simulink library "dotFinder_ul"  (R2018b)
settings: Solver=VariableStepAuto  StartTime=0.0  StopTime=10.0  RelTol=1e-3
libraries: simulink x2
settings Model: Creator=mcobb  LastModifiedBy=mcobb
settings DebuggingCC: LibraryContextMissingDiagnostic=none
settings SFSimCC: SimUseLocalCustomCode=off
settings RTWCC: RTWUseLocalCustomCode=off

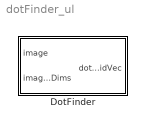
== system dotFinder_ul ==
  DotFinder : Subsystem  mask{ROIPositionHoldEnable=on, ROIPositionHoldCoordinates=1*[500 500], ROIDimVec_px=[40 100], ImageDimensions=[1000 2000]}
      mask prompts: ROIPositionHoldEnable "Hold Position Enable"; ROIPositionHoldCoordinates "Hold Position Coordinates  [rows cols]  (pixels)"; ROIDimVec_px "Dimensions [rows cols]  (pixels)"; ImageDimensions "Image Dimensions [rows cols] in pixels"
      mask DialogControl ParameterGroupVar Prompt: Region Of Interest (ROI) Parameters
      mask DialogControl Container3 Prompt: Other Parameters

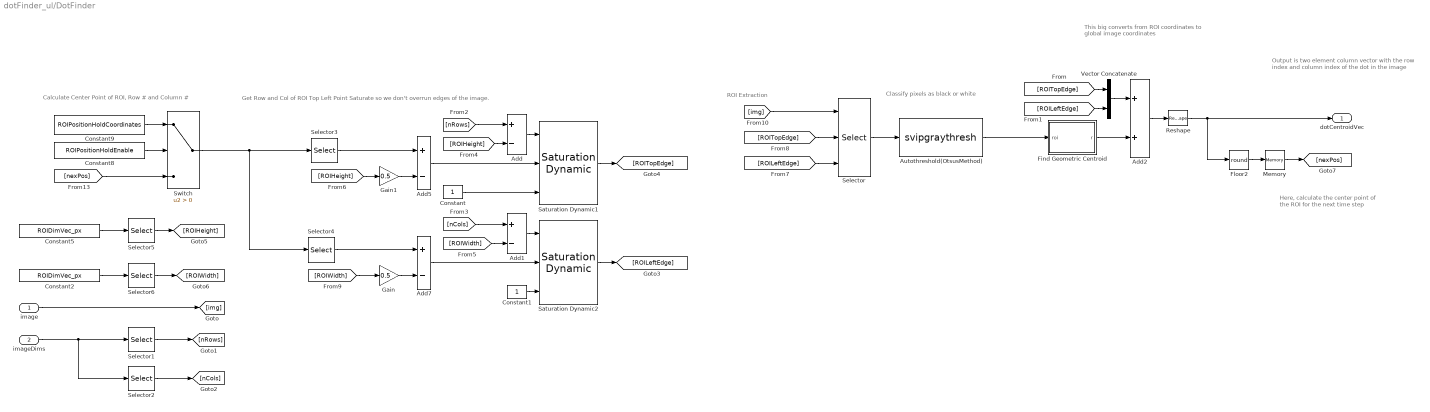
== system dotFinder_ul/DotFinder ==
  note: This big converts from ROI coordinates
      | to global image coordinates
  note: Here, calculate the center point of
      | the ROI for the next time step
  note: Output is two element column vector with the row
      | index and column index of the dot in the image
  note: Classify pixels as black or white
  note: Get Row and Col of ROI Top Left Point
      | Saturate so we don't overrun edges of the image.
  note: Calculate Center Point of ROI, Row # and Column #
  note: ROI Extraction
  image : Inport
  imageDims : Inport  Port=2
  Add{,1,5,7} (4 alike) : Sum  Inputs=+-
  Add2 : Sum
  Autothreshold(OtsusMethod) : S-Function  DialogController=vipDDGCreate  FunctionName=svipgraythresh  Parameters=operator, userDefinedRange, umin, umax, threshOut, effMetricOut, outOfRngOpt, scaleThreshold, scaleFactor, P1Mode, P1WordLength, P1FracLength, A1Mode, A1WordLength, A1FracLength, P2Mode, P2WordLength, P2FracLength, A2Mode, A2WordLength, A2FracLength, P3Mode, P3WordLength, P3FracLength, A3Mode, A3WordLength, A3FracLength, P4Mode, P4WordLength, P4FracLength, A4Mode, A4WordLength, A4FracLength, Q1Mode, Q1WordLength, Q1FracLength, EMMode, EMWordLength, EMFracLength, dtInfo.roundingMode, dtInfo.overflowMode  SFunctionDeploymentMode=off  EnableBusSupport=off  mask(Autothreshold){operator=>, threshOut=off, effMetricOut=off, userDefinedRange=off, umin=0, umax=255, outOfRngOpt=Ignore, scaleThreshold=off, scaleFactor=1, P1Mode=Specify word length, P1WordLength=32, P1FracLength=30, A1Mode=Same as Product 1, A1WordLength=32, A1FracLength=30, P2Mode=Specify word length, P2WordLength=32, P2FracLength=22, A2Mode=Same as Product 2, A2WordLength=32, A2FracLength=22, P3Mode=Specify word length, P3WordLength=32, P3FracLength=14, A3Mode=Same as Product 3, A3WordLength=32, A3FracLength=14, P4Mode=Binary point scaling, P4WordLength=32, P4FracLength=15, A4Mode=Same as Product 4, A4WordLength=16, A4FracLength=4, Q1Mode=Specify word length, Q1WordLength=32, Q1FracLength=16, EMMode=Specify word length, EMWordLength=16, EMFracLength=14, roundingMode=Floor, overflowMode=off, LockScale=off}
      mask prompts: operator "vision:masks:ThresholdingOperator"; threshOut "vision:masks:OutputThreshold"; effMetricOut "vision:masks:OutputEffectivenessMetric"; userDefinedRange "vision:masks:SpecifyDataRange"; umin "vision:masks:MinimumValueOfInput"; umax "vision:masks:MinimumValueOfInput"; outOfRngOpt "vision:masks:WhenDataRangeIsExceeded"; scaleThreshold "vision:masks:ScaleThreshold_MP"; scaleFactor "vision:masks:ThresholdScalingFactor"; P1Mode "P1:"; P1WordLength "P1 WL:"; P1FracLength "P1 FL:"; A1Mode "A1:"; A1WordLength "A1 WL:"; A1FracLength "A1 FL:"; P2Mode "P2:"; P2WordLength "P2 WL:"; P2FracLength "P2 FL:"; A2Mode "A2:"; A2WordLength "A2 WL:"; A2FracLength "A2 FL:"; P3Mode "P3:"; P3WordLength "P3 WL:"; P3FracLength "P3 FL:"; A3Mode "A3:"; A3WordLength "A3 WL:"; A3FracLength "A3 FL:"; P4Mode "P4:"; P4WordLength "P4 WL:"; P4FracLength "P4 FL:"; A4Mode "A4:"; A4WordLength "A4 WL:"; A4FracLength "A4 FL:"; Q1Mode "Q1:"; Q1WordLength "Q1 WL:"; Q1FracLength "Q1 FL:"; EMMode "EM:"; EMWordLength "EM WL:"; EMFracLength "EM FL:"; roundingMode "vision:masks:RoundIntegerCalculationsTowards"; overflowMode "vision:masks:RoundIntegerCalculationsTowards"; LockScale "vision:masks:LockScaling"
      mask help: vision:masks:AutoThresholdDescription
      mask init:
      | blk = gcbh;
      | 
      | dtInfo = dspGetFixptDataTypeInfo(blk,1);
      | 
      | effMetricOut_str = get_param(blk,'effMetricOut');
      | threshOut_str = get_param(blk,'threshOut');
      | if strcmp(effMetricOut_str,'off') && strcmp(threshOut_str,'off')
      | 	[so(1:3).port] = deal(1,1,1);
      | 	[so(1:3).txt] = deal('BW','BW','BW');
      | elseif strcmp(effMetricOut_str,'on') && strcmp(threshOut_str,'off')
      | 	[so(1:3).port] = deal(1,2,2);
      | 	[so(1:3).txt] = deal('BW','EMetric','EMetric');
      | elseif strcmp(effMetricOut_str,'off') && strcmp(threshOut_str,'on')
      | 	[so(1:3).port] = deal(1,2,2);
      | 	[so(1:3).txt] = deal('BW','Th','Th');
      | else
      | 	[so(1:3).port] = deal(1,2,3);
      | 	[so(1:3).txt] = deal('BW','Th','EMetric');
      | end
      mask Help: eval('visionblockhelp');
      mask TypeOptions operator: > | <=
      mask TypeOptions outOfRngOpt: vision:masks:Ignore | vision:masks:Saturate | vision:masks:WarnAndSaturate | vision:masks:Error
      mask TypeOptions P1Mode: Specify word length | Binary point scaling | Slope and bias scaling
      mask TypeOptions A1Mode: Same as Product 1 | Specify word length | Binary point scaling | Slope and bias scaling
      mask TypeOptions P2Mode: Specify word length | Binary point scaling | Slope and bias scaling
      mask TypeOptions A2Mode: Same as Product 2 | Specify word length | Binary point scaling | Slope and bias scaling
      mask TypeOptions P3Mode: Specify word length | Binary point scaling | Slope and bias scaling
      mask TypeOptions A3Mode: Same as Product 3 | Specify word length | Binary point scaling | Slope and bias scaling
      mask TypeOptions P4Mode: Same as input | Binary point scaling | Slope and bias scaling
      mask TypeOptions A4Mode: Same as Product 4 | Binary point scaling | Slope and bias scaling
      mask TypeOptions Q1Mode: Specify word length | Binary point scaling | Slope and bias scaling
      mask TypeOptions EMMode: Specify word length | Binary point scaling | Slope and bias scaling
      mask TypeOptions roundingMode: dspshared:FixptDialog:Ceiling_CB | dspshared:FixptDialog:Convergent_CB | dspshared:FixptDialog:Floor_CB | dspshared:FixptDialog:Nearest_CB | dspshared:FixptDialog:Round_CB | dspshared:FixptDialog:Simplest_CB | dspshared:FixptDialog:Zero_CB
      mask Display:
      | disp('Autothreshold');
      | port_label('input',1,'I');
      | port_label('output',so(1).port, so(1).txt);
      | port_label('output',so(2).port, so(2).txt);
      | port_label('output',so(3).port, so(3).txt);
  Constant : Constant
  Constant1 : Constant
  Constant2 : Constant  Value=ROIDimVec_px
  Constant5 : Constant  Value=ROIDimVec_px
  Constant8 : Constant  Value=ROIPositionHoldEnable
  Constant9 : Constant  Value=ROIPositionHoldCoordinates
  Find Geometric Centroid : MATLAB Function  TreatAsAtomicUnit=on
  Floor2 : Rounding  Operator=round
  Gain : Gain  Gain=0.5
  Gain1 : Gain  Gain=0.5
  Memory : Memory  InitialCondition=ROIPositionHoldCoordinates(:)
  Reshape : Reshape  OutputDimensionality=Column vector (2-D)
  Saturation Dynamic1 : simulink/Discontinuities/Saturation Dynamic  OutMin=[]  OutMax=[]  OutDataTypeStr=Inherit: Same as second input  OutDataType=fixdt(1, 16)  OutScaling=2^-10  DoSatur=off
  Saturation Dynamic2 : simulink/Discontinuities/Saturation Dynamic  OutMin=[]  OutMax=[]  OutDataTypeStr=Inherit: Same as second input  OutDataType=fixdt(1, 16)  OutScaling=2^-10  DoSatur=off
  Selector : Selector  NumberOfDimensions=2  InputPortWidth=3  IndexOptions=Starting index (port),Starting index (port)  Indices=[1 3],1  OutputSizes=ROIDimVec_px(1),ROIDimVec_px(2)
  Selector1 : Selector  InputPortWidth=2  IndexOptions=Index vector (dialog)  Indices=1  OutputSizes=1
  Selector2 : Selector  InputPortWidth=2  IndexOptions=Index vector (dialog)  Indices=2  OutputSizes=1
  Selector3 : Selector  InputPortWidth=2  IndexOptions=Index vector (dialog)  Indices=1  OutputSizes=1
  Selector4 : Selector  InputPortWidth=2  IndexOptions=Index vector (dialog)  Indices=2  OutputSizes=1
  Selector5 : Selector  InputPortWidth=2  IndexOptions=Index vector (dialog)  Indices=1  OutputSizes=1
  Selector6 : Selector  InputPortWidth=2  IndexOptions=Index vector (dialog)  Indices=2  OutputSizes=1
  Switch : Switch  Criteria=u2 > Threshold
  Vector Concatenate : Concatenate
  dotCentroidVec : Outport  PortDimensions=[2 1]
  wires:
  Add2/1 -> Reshape/1
  Find Geometric Centroid/1(r) -> Add2/2
  Vector Concatenate/1 -> Add2/1
  [ROITopEdge] -> Vector Concatenate/1
  [ROILeftEdge] -> Vector Concatenate/2
  Switch/1 -> Selector4/1, Selector3/1
  Gain1/1 -> Add5/2
  Gain/1 -> Add7/2
  [img] -> Selector/1
  Selector3/1 -> Add5/1
  Selector4/1 -> Add7/1
  Add5/1 -> Saturation Dynamic1/2
  [ROILeftEdge] -> Selector/3
  [ROITopEdge] -> Selector/2
  Selector/1 -> Autothreshold(OtsusMethod)/1
  image/1 -> [img]
  Selector1/1 -> [nRows]
  Selector2/1 -> [nCols]
  Selector6/1 -> [ROIWidth]
  Selector5/1 -> [ROIHeight]
  Constant5/1 -> Selector5/1
  Saturation Dynamic1/1 -> [ROITopEdge]
  Constant/1 -> Saturation Dynamic1/3
  Constant1/1 -> Saturation Dynamic2/3
  Add7/1 -> Saturation Dynamic2/2
  Saturation Dynamic2/1 -> [ROILeftEdge]
  Add/1 -> Saturation Dynamic1/1
  [ROIHeight] -> Add/2
  [nRows] -> Add/1
  Add1/1 -> Saturation Dynamic2/1
  [nCols] -> Add1/1
  [ROIWidth] -> Add1/2
  [ROIHeight] -> Gain1/1
  [ROIWidth] -> Gain/1
  Autothreshold(OtsusMethod)/1 -> Find Geometric Centroid/1(roi)
  Constant2/1 -> Selector6/1
  Memory/1 -> [nexPos]
  Constant8/1 -> Switch/2
  Constant9/1 -> Switch/1
  [nexPos] -> Switch/3
  Floor2/1 -> Memory/1
  imageDims/1 -> Selector2/1, Selector1/1
  Reshape/1 -> Floor2/1, dotCentroidVec/1

== matlab function dotFinder_ul/DotFinder/Find Geometric Centroid ==
  data: roi input; r output size=[2 1]
function r = fcn(roi)
% Function to calculate row and column index of the geometric centroid of
% the ROI.

% Total number of white pixels
N = sum(sum(roi));

% r = [rowIndex colIndex]^T
r = [([1:size(roi,1)]*sum(roi,2))/N;...
     ([1:size(roi,2)]*sum(roi,1)')/N];
